simulink model "CLmodel"  (R2018b)
settings: Solver=VariableStepAuto  StartTime=0.0  StopTime=10.0  RelTol=1e-3
values from neighbouring files (symbols this model uses):
  I = 1    [essai_Noncolocated.m]
  I_f_C = 0    [essai_Noncolocated.m]
  I_tot_P = inv(dcgain(G(4,4)))    [essai_Noncolocated.m]
libraries: cstblocks x2
settings Model: Creator=d.alazard  LastModifiedBy=d.alazard

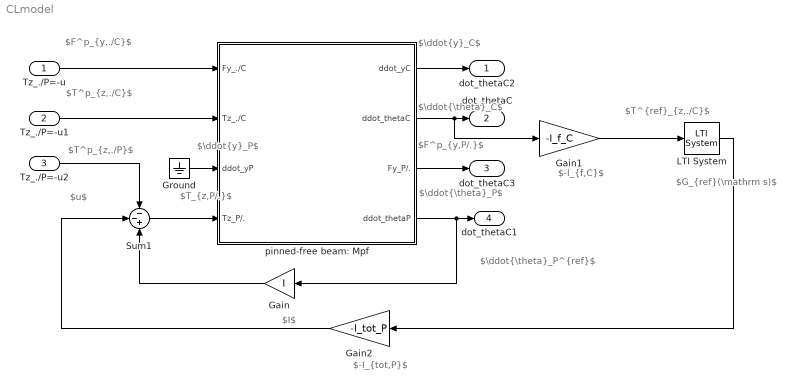
== system CLmodel ==
  note: $G_{ref}(\mathrm s)$
  note: $-I_{f,C}$
  note: $\ddot{y}_P$
  note: $\ddot{\theta}_P$
  note: $\ddot{\theta}_C$
  note: $u$
  note: $T^p_{z,./P}$
  note: $T^p_{z,./C}$
  note: $F^p_{y,./C}$
  note: $F^p_{y,P/.}$
  note: $\ddot{y}_C$
  note: $T_{z,P/.}$
  note: $I$
  note: $\ddot{\theta}_P^{ref}$
  note: $T^{ref}_{z,./C}$
  note: $-I_{tot,P}$
  Tz_./P=-u : Inport
  Tz_./P=-u1 : Inport  Port=2
  Tz_./P=-u2 : Inport  Port=3
  Gain : Gain  Gain=I
  Gain1 : Gain  Gain=-I_f_C
  Gain2 : Gain  Gain=-I_tot_P
  Ground : Ground
  LTI System : cstblocks/LTI System  sys=Gref  IC=[]
  Sum1 : Sum  Inputs=--+
  pinned-free beam: Mpf : Subsystem
  dot_thetaC2 : Outport
  dot_thetaC : Outport  Port=2
  dot_thetaC3 : Outport  Port=3
  dot_thetaC1 : Outport  Port=4
  wires:
  Tz_./P=-u/1 -> pinned-free beam: Mpf/1(Fy_./C)
  Tz_./P=-u1/1 -> pinned-free beam: Mpf/2(Tz_./C)
  Ground/1 -> pinned-free beam: Mpf/3(ddot_yP)
  Sum1/1 -> pinned-free beam: Mpf/4(Tz_P/.)
  pinned-free beam: Mpf/3(Fy_P/.) -> dot_thetaC3/1
  pinned-free beam: Mpf/1(ddot_yC) -> dot_thetaC2/1
  pinned-free beam: Mpf/2(ddot_thetaC) -> Gain1/1, dot_thetaC/1
  pinned-free beam: Mpf/4(ddot_thetaP) -> dot_thetaC1/1, Gain/1
  Gain/1 -> Sum1/3
  Tz_./P=-u2/1 -> Sum1/1
  Gain2/1 -> Sum1/2
  Gain1/1 -> LTI System/1
  LTI System/1 -> Gain2/1

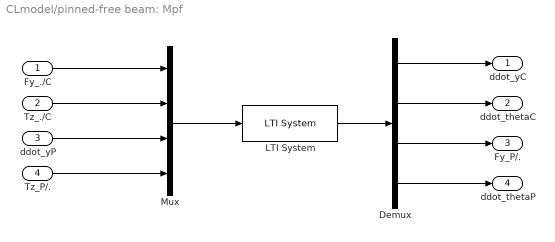
== system CLmodel/pinned-free beam: Mpf ==
  Fy_./C : Inport
  Tz_./C : Inport  Port=2
  ddot_yP : Inport  Port=3
  Tz_P/. : Inport  Port=4
  Demux : Demux
  LTI System : cstblocks/LTI System  sys=Mpf  IC=[]
  Mux : Mux
  ddot_yC : Outport
  ddot_thetaC : Outport  Port=2
  Fy_P/. : Outport  Port=3
  ddot_thetaP : Outport  Port=4
  wires:
  Tz_./C/1 -> Mux/2
  Demux/4 -> ddot_thetaP/1
  Demux/1 -> ddot_yC/1
  Tz_P/./1 -> Mux/4
  Demux/3 -> Fy_P/./1
  Fy_./C/1 -> Mux/1
  Demux/2 -> ddot_thetaC/1
  ddot_yP/1 -> Mux/3
  LTI System/1 -> Demux/1
  Mux/1 -> LTI System/1
